simulink model "deltasigma2"  (Simulink 7.6)
settings: Solver=ode45  StartTime=0  StopTime=10  MaxStep=1/2048  RelTol=1e-3
libraries: simeventssignalmanage1 x4, dsparch4 x1, simulink_extras x1, simulink x1
settings Model: Creator=Robin  LastModifiedBy=Robin
settings SimEventsCC: propDiagAttribOutput=1  propDiagFcnCallOutput=1  propDiagStatOutput=0

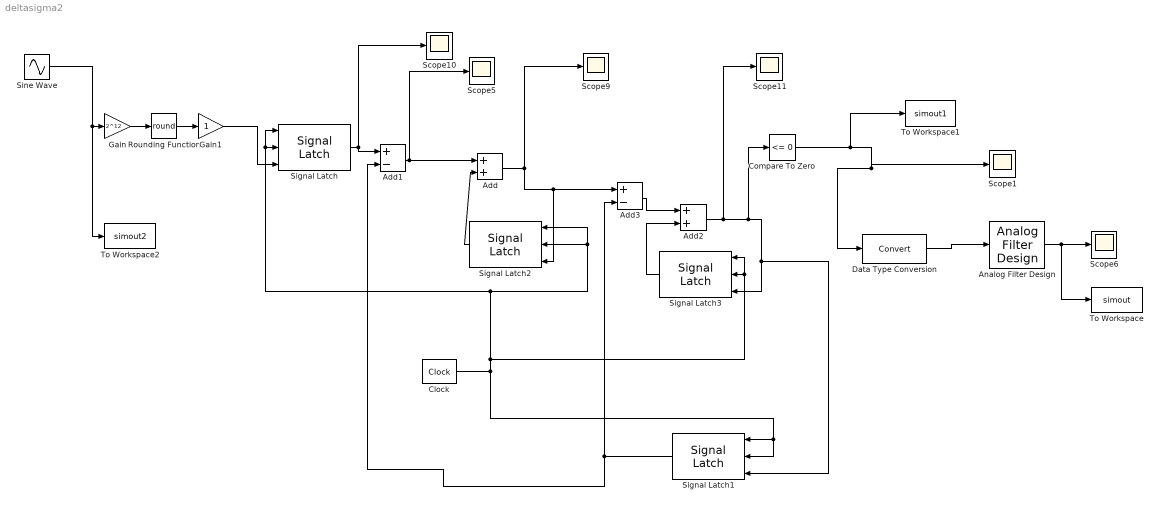
== system deltasigma2 ==
  Add : Sum  AccumDataTypeStr=int16  RndMeth=Convergent
  Add1 : Sum  Inputs=+-  AccumDataTypeStr=int16  RndMeth=Nearest
  Add2 : Sum  AccumDataTypeStr=int16  RndMeth=Convergent
  Add3 : Sum  Inputs=+-  AccumDataTypeStr=int16  RndMeth=Convergent
  Analog Filter Design : dsparch4/Analog Filter Design  method=Butterworth  filttype=Bandpass  N=2  Wlo=1  Whi=10*pi  Rp=2  Rs=40
  Clock : simulink_extras/Flip Flops/Clock  SystemSampleTime=-1  period=1/400
  Compare To Zero : simulink/Logic and Bit Operations/Compare To Zero  SystemSampleTime=-1  relop=<=  LogicOutDataTypeMode=uint8
  Data Type Conversion : DataTypeConversion  RndMeth=Convergent
  Gain : Gain  Gain=2^12
  Gain1 : Gain
  Rounding Function : Rounding  Operator=round
  Scope{1,5..6,9..11} (6 alike) : Scope
      Scope10 settings: SaveName=ScopeData9
      Scope11 settings: SaveName=ScopeData10
      Scope5 settings: SaveName=ScopeData3
      Scope6 settings: TimeRange=1  YMin=-0.5  YMax=1.5  SaveName=ScopeData5
      Scope9 settings: SaveName=ScopeData7
  Signal Latch{,1..3} (4 alike) : simeventssignalmanage1/Signal Latch  SystemSampleTime=-1  InitialMemoryValue=0  WriteMemoryUpon=Change in signal from port wvc  MemoryWriteEdgeOption=Rising  SpecifyWriteEventPriority=on  PriorityMemoryWrite=7100  ReadMemoryUpon=Change in signal from port rvc  MemoryReadEdgeOption=Falling  SpecifyReadEventPriority=on  PriorityMemoryRead=7000  ReportMemoryState=off  ReportMemoryUponWrite=off  ReportMemoryUponRead=on
  Sine Wave : Sin  Frequency=3*pi  SampleTime=0
  To Workspace : ToWorkspace  VariableName=simout  SampleTime=-1  SaveFormat=Structure With Time
  To Workspace1 : ToWorkspace  VariableName=simout1  SampleTime=-1  SaveFormat=Structure With Time
  To Workspace2 : ToWorkspace  VariableName=simout2  SampleTime=-1  SaveFormat=Structure With Time
  wires:
  Signal Latch/1 -> Add1/1, Scope10/1
  Signal Latch2/1 -> Add/2
  Clock/1 -> Signal Latch2/2, Signal Latch2/1, Signal Latch/1, Signal Latch/2, Signal Latch1/1, Signal Latch1/2, Signal Latch3/2, Signal Latch3/1
  Signal Latch1/1 -> Add3/2, Add1/2
  Analog Filter Design/1 -> To Workspace/1, Scope6/1
  Signal Latch3/1 -> Add2/2
  Add2/1 -> Scope11/1, Signal Latch3/3, Signal Latch1/3, Compare To Zero/1
  Add3/1 -> Add2/1
  Add1/1 -> Scope5/1, Add/1
  Gain/1 -> Rounding Function/1
  Rounding Function/1 -> Gain1/1
  Sine Wave/1 -> Gain/1, To Workspace2/1
  Add/1 -> Signal Latch2/3, Add3/1, Scope9/1
  Compare To Zero/1 -> Data Type Conversion/1, Scope1/1, To Workspace1/1
  Data Type Conversion/1 -> Analog Filter Design/1
  Gain1/1 -> Signal Latch/3
